simulink model "triggers"  (R2023b)
settings: Solver=VariableStepAuto  StartTime=0.0  StopTime=10.0  RelTol=1e-3
settings Model: Creator=1234  LastModifiedBy=1234

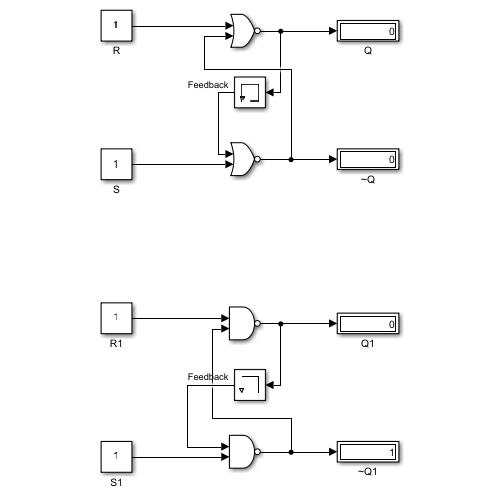
[thumbnail: Simulink's stored preview of the top-level diagram]
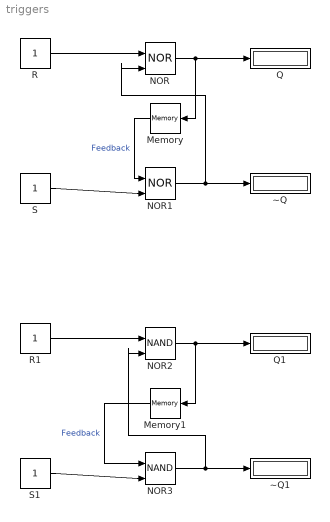
== system triggers ==
  Memory : Memory
  Memory1 : Memory
  NOR : Logic  Operator=NOR  IconShape=distinctive  AllPortsSameDT=off  OutDataTypeStr=boolean
  NOR1 : Logic  Operator=NOR  IconShape=distinctive  AllPortsSameDT=off  OutDataTypeStr=boolean
  NOR2 : Logic  Operator=NAND  IconShape=distinctive  AllPortsSameDT=off  OutDataTypeStr=boolean
  NOR3 : Logic  Operator=NAND  IconShape=distinctive  AllPortsSameDT=off  OutDataTypeStr=boolean
  Q : Display
  Q1 : Display
  R : Constant
  R1 : Constant
  S : Constant
  S1 : Constant
  ~Q : Display
  ~Q1 : Display
  wires:
  S/1 -> NOR1/2
  R/1 -> NOR/1
  NOR/1 -> Q/1, Memory/1
  NOR1/1 -> NOR/2, ~Q/1
  Memory/1 -> NOR1/1  "Feedback"
  Memory1/1 -> NOR3/1  "Feedback"
  NOR3/1 -> ~Q1/1, NOR2/2
  NOR2/1 -> Memory1/1, Q1/1
  R1/1 -> NOR2/1
  S1/1 -> NOR3/2
